simulink model "TestNetwork_SPDN2_AllWires"  (R2014b)
settings: Solver=FixedStepDiscrete  StartTime=0.0  StopTime=100  FixedStep=1  RelTol=1e-3
InitFcn:
  | initialize;
StopFcn:
  | OutputPlotting;
libraries: BlockLib x13, dspsrcs4 x1
settings Model: Creator=kunalmenda  LastModifiedBy=kunalmenda
settings SolverCC: AlgebraicLoopSolver=LineSearch

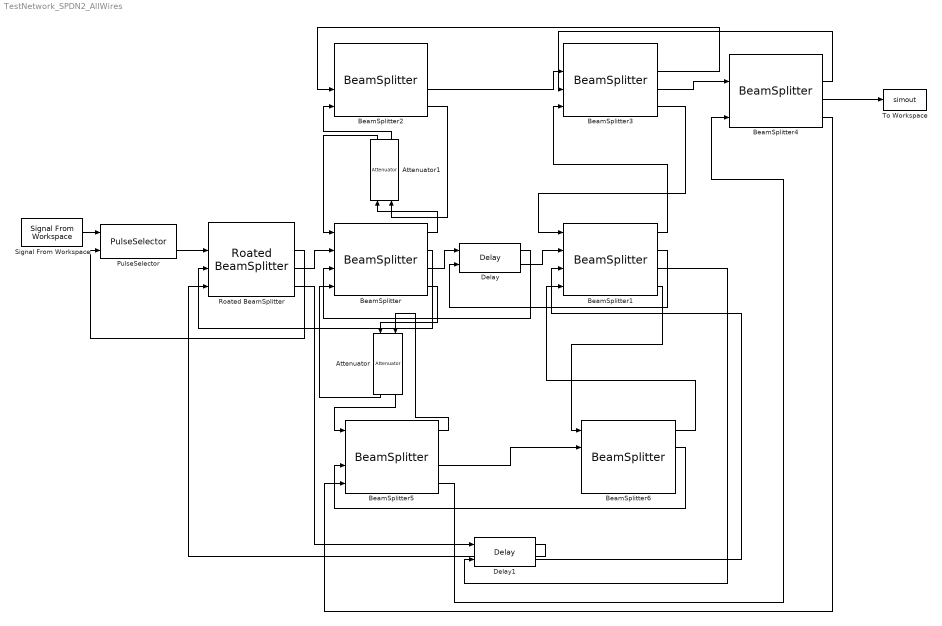
== system TestNetwork_SPDN2_AllWires ==
  Attenuator : BlockLib/Attenuator  AttnFactor=0.5
  Attenuator1 : BlockLib/Attenuator  AttnFactor=0.5
  BeamSplitter{,1..6} (7 alike) : BlockLib/BeamSplitter  Transmittance=0.50  Reflectance=0.50  Ghost=0.01  BackReflectance=0.001
  Delay : BlockLib/Delay  DelayAmt=0.2e-7
  Delay1 : BlockLib/Delay  DelayAmt=0.6e-7
  PulseSelector : BlockLib/PulseSelector  PCTimings=[-1,1]*1e-9  ControlPowers=[1.0]
  Roated BeamSplitter : BlockLib/Roated BeamSplitter  Transmittance=0.50  Reflectance=0.50  Ghost=0.01  BackReflectance=0.001
  Signal From Workspace : dspsrcs4/Signal From Workspace  X=inputsignal  Ts=1  nsamps=1  OutputAfterFinalValue=Setting to zero  ignoreOrWarnInputAndFrameLengths=off
  To Workspace : ToWorkspace  VariableName=simout  SaveFormat=Timeseries  SampleTime=-1
  wires:
  Signal From Workspace/1 -> PulseSelector/1
  PulseSelector/2 -> Roated BeamSplitter/2
  Roated BeamSplitter/3 -> BeamSplitter/2
  BeamSplitter/3 -> Delay/1
  Delay/2 -> BeamSplitter1/2
  BeamSplitter1/1 -> BeamSplitter3/4
  BeamSplitter/1 -> Attenuator1/1
  Attenuator1/2 -> BeamSplitter2/4
  BeamSplitter/4 -> Attenuator/1
  Attenuator/2 -> BeamSplitter5/1
  BeamSplitter2/3 -> BeamSplitter3/2
  BeamSplitter3/3 -> BeamSplitter4/2
  Roated BeamSplitter/4 -> Delay1/1
  Delay1/2 -> BeamSplitter1/3
  BeamSplitter5/4 -> BeamSplitter4/4
  BeamSplitter4/3 -> To Workspace/1
  BeamSplitter1/2 -> Delay/2
  Delay/1 -> BeamSplitter/3
  BeamSplitter1/4 -> BeamSplitter6/1
  BeamSplitter6/2 -> BeamSplitter5/3
  BeamSplitter4/4 -> BeamSplitter5/4
  BeamSplitter5/3 -> BeamSplitter6/2
  BeamSplitter6/1 -> BeamSplitter1/4
  BeamSplitter/2 -> Roated BeamSplitter/3
  Roated BeamSplitter/2 -> PulseSelector/2
  Delay1/1 -> Roated BeamSplitter/4
  BeamSplitter1/3 -> Delay1/2
  BeamSplitter5/1 -> Attenuator/2
  Attenuator/1 -> BeamSplitter/4
  Attenuator1/1 -> BeamSplitter/1
  BeamSplitter2/4 -> Attenuator1/2
  BeamSplitter3/2 -> BeamSplitter2/3
  BeamSplitter4/2 -> BeamSplitter3/3
  BeamSplitter3/4 -> BeamSplitter1/1
